simulink model "black_box_ex1_new"  (Simulink 7.3)
settings: Solver=VariableStepDiscrete  SolverMode=SingleTasking  StartTime=0.0  StopTime=500  RelTol=1e-3
undefined symbols (not defined in the file or in its folder): dfilt, xlipgetpartsetting
libraries: xbsIndex_r4 x12, xbsCopyrightNotice_r4 x1, dsparch4 x1, dspobslib x1, simulink x1
settings Model: Creator=alexc  LastModifiedBy=douangp
settings DataIOCC: SignalLoggingName=sigsOut
settings OptimizationCC: InitFltsAndDblsToZero=on
settings DebuggingCC: SaveWithParameterizedLinksMsg=none  SignalResolutionControl=TryResolveAllWithWarning  SolverPrmCheckMsg=none  MultiTaskDSMMsg=warning  MultiTaskCondExecSysMsg=none  StrictBusMsg=None
settings HardwareCC: TargetUnknown=on
settings RTWCC: IncludeERTFirstTime=on
settings GRTTargetCC: TargetFcnLib=ansi_tfl_tmw.mat

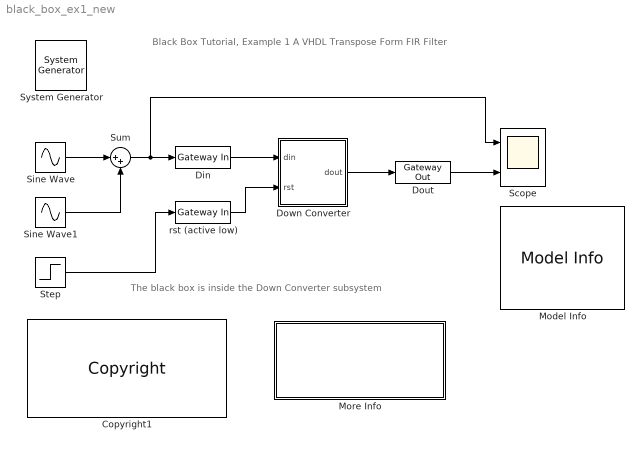
== system black_box_ex1_new ==
  note: Black Box Tutorial, Example 1
      | A VHDL Transpose Form FIR Filter
  note: The black box is inside the
      | Down Converter subsystem
  " System Generator" : xbsIndex_r4/ System Generator  Tag=genX  SystemSampleTime=-1  xilinxfamily=virtex6  part=xc6vlx240t  speed=-1  package=ff1156  synthesis_tool=XST  clock_wrapper=Clock Enables  directory=./netlist  testbench=off  simulink_period=1  sysclk_period=5  dcm_input_clock_period=100  incr_netlist=off  trim_vbits=Everywhere in SubSystem  dbl_ovrd=According to Block Masks  core_generation=According to Block Masks  run_coregen=off  deprecated_control=off  eval_field=0  block_type=sysgen
      settings: block_version=9.2.01
  Copyright1 : xbsCopyrightNotice_r4/Copyright  copyrighttext="Copyright (c) 2009  by  Xilinx, Inc. All rights reserved.<br><br>This file contains proprietary, confidential information of Xilinx, Inc., is distributed under licensefrom Xilinx, Inc., and may be used, copied and/or disclosed only pursuant to the terms of a valid licenseagreement with Xilinx, Inc. Xilinx hereby grants you a license to use this file solely for design,simulation, implementation and creation of design files limited to Xilinx devices or technologies. Use with non-Xilinx devices or technologies is expressly prohibited and immediately terminates your license unless covered by a separate agreement.<br><br>Xilinx is providing this design, code, or information \"as-is\" solely for use in developing programs and solutions for Xilinx devices, with no obligation on the part of Xilinx to provide support. By providingthis design, code, or information as one possible implementation of this feature, application or standard,Xilinx is making no representation that this implementation is free from any claims of infringement. Youare responsible for obtaining any rights you may require for your implementation. Xilinx expressly disclaimsany warranty whatsoever with respect to the adequacy of the implementation, including but not limited to anywarranties or representations that this implementation is free from claims of infringement, implied warrantiesof merchantability or fitness for a particular purpose.<br><br>Xilinx products are not intended for use in life support appliances, devices, or systems. Use in such applications is expressly prohibited.<br><br>Any modifications that are made to the Source Code are done at the user's sole risk and will be unsupported.<br><br>This copyright and support notice must be retained as part of this text at all times. (c) Copyright 1995-2009 Xilinx, Inc. All rights reserved."  block_type=copyright
      settings: block_version=10.1.00
      settings: infoedit=|
      | Copyright(C) 2008 by  Xilinx, Inc. All rights reserved.<br>
      | <br>
      | This file contains proprietary, confidential information of Xilinx, Inc., is distributed under license
      | from Xilinx, Inc., and may be used, copied and/or disclosed only pursuant to the terms of a valid license
      | agreement with Xilinx, Inc. Xilinx hereby grants you a license to use this file solely for design,
      | simulation, implementation and creation of design files limited to Xilinx devices or technologies. Use
      | with non-Xilinx devices or technologies is expressly prohibited and immediately terminates your license
      | unless covered by a separate agreement.<br>
      | <br>
      | Xilinx is providing this design, code, or information "as-is" solely for use in developing programs and
      | solutions for Xilinx devices, with no obligation on the part of Xilinx to provide support. By providing
      | this design, code, or information as one possible implementation of this feature, application or standard,
      | Xilinx is making no representation that this implementation is free from any claims of infringement. You
      | are responsible for obtaining any rights you may require for your implementation. Xilinx expressly disclaims
      | any warranty whatsoever with respect to the adequacy of the implementation, including but not limited to any
      | warranties or representations that this implementation is free from claims of infringement, implied warranties
      | of merchantability or fitness for a particular purpose.<br>
      | <br>
      | Xilinx products are not intended for use in life support appliances, devices, or systems. Use in such
      | applications is expressly prohibited.<br>
      | <br>
      | Any modifications that are made to the Source Code are done at the user's sole risk and will be unsupported.<br>
      | <br>
      | This copyright and support notice must be retained as part of this text at all times.
      | (c) Copyright 1995-2008 Xilinx, Inc. All rights reserved.
  Din : xbsIndex_r4/Gateway In  arith_type="Signed  (2's comp)"  n_bits=10  bin_pt=8  quantization="Round  (unbiased: +/- Inf)"  overflow=Saturate  period=1  dbl_ovrd=off  timing_constraint=None  locs_specified=off  LOCs={}  block_type=gatewayin
      settings: infoedit="Gateway in block.  Converts inputs of type Simulink integer, double and fixed point to  Xilinx fixed point type.<P><P>Hardware notes:  In hardware these blocks become top level input ports."  xl_area=[0, 0, 0, 0, 0, 0, 0]  block_version=VER_STRING_GOES_HERE
  Dout : xbsIndex_r4/Gateway Out  hdl_port=on  timing_constraint=None  locs_specified=off  LOCs={}  block_type=gatewayout
      settings: infoedit="Gateway out block.  Converts Xilinx fixed point inputs into ouputs of type Simulink integer, double, or fixed point.<P><P>Hardware notes:  In hardware these blocks become top level output ports or are discarded, depending on how they are configured."  xl_area=[0, 0, 0, 0, 0, 0, 0]  block_version=VER_STRING_GOES_HERE
  Down Converter : Subsystem
  Model Info : simulink/Model-Wide Utilities/Model Info  SystemSampleTime=-1  InitialBlockCM=None  BlockCM=None  Frame=on  DisplayStringWithTags=|  HorizontalTextAlignment=Left  LeftAlignmentValue=0.02  SourceBlockDiagram=black_box_ex1_new  TagMaxNumber=20
      | Model Info
      | Created by %<Created>
      | Modified by %<ModifiedBy>
      | Model version %<ModelVersion>
  More Info : Subsystem
      settings: OpenFcn=xlDoc('-book','sysgen', '-title', 'Black Box');
      mask Display: disp('Double click\n for System Generator\n documentation on\n related topics.')
  Scope : Scope  NumInputPorts=2
      settings: YMin=-2~-7000  YMax=2~7000
  Sine Wave : Sin  Amplitude=1  Bias=0  Frequency=2*pi*.31  Phase=0  Samples=10  SampleTime=1  Offset=0
  Sine Wave1 : Sin  Amplitude=1  Bias=0  Frequency=2*pi*.45  Phase=0  Samples=10  SampleTime=1  Offset=0
  Step : Step  SampleTime=1
  Sum : Sum  Inputs=|++  OutDataType=sfix(16)  OutScaling=2^0  SaturateOnIntegerOverflow=on
  rst (active low) : xbsIndex_r4/Gateway In  arith_type=Boolean  n_bits=10  bin_pt=8  quantization="Round  (unbiased: +/- Inf)"  overflow=Saturate  period=1  dbl_ovrd=off  timing_constraint=None  locs_specified=off  LOCs={}  block_type=gatewayin
      settings: infoedit="Gateway in block.  Converts inputs of type Simulink integer, double and fixed point to  Xilinx fixed point type.<P><P>Hardware notes:  In hardware these blocks become top level input ports."  xl_area=[0, 0, 0, 0, 0, 0, 0]  block_version=VER_STRING_GOES_HERE
  wires:
  Down Converter/1(dout) -> Dout/1
  Din/1 -> Down Converter/1(din)
  Dout/1 -> Scope/2
  Sine Wave/1 -> Sum/1
  Sine Wave1/1 -> Sum/2
  Sum/1 -> Din/1, Scope/1
  rst (active low)/1 -> Down Converter/2(rst)
  Step/1 -> rst (active low)/1

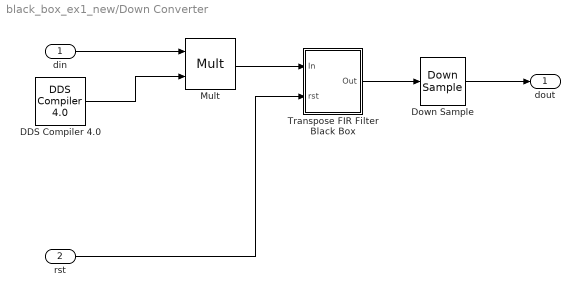
== system black_box_ex1_new/Down Converter ==
  din : Inport  OutDataType=sfix(16)  OutScaling=2^0
  rst : Inport  Port=2  OutDataType=sfix(16)  OutScaling=2^0
  "DDS Compiler 4.0 " : xbsIndex_r4/DDS Compiler 4.0   partspresent=Phase_Generator_and_SIN_COS_LUT  dds_clock_rate=100  channels=1  parameter_entry=System_Parameters  spurious_free_dynamic_range=50  frequency_resolution=0.4  noise_shaping=None  phase_width=28  output_width=6  output_selection=Sine  negative_sine=off  negative_cosine=off  amplitude_mode=Full_Range  memory_type=Auto  optimization_goal=Auto  dsp48_use=Minimal  latency_configuration=Auto  latency=2  has_phase_out=off  sclr_pin=off  clock_enable=off  rfd=off  rdy=off  channel_pin=off  explicit_period=on  period=1  phase_increment=Fixed  output_frequency1=30  output_frequency2=0  output_frequency3=0  output_frequency4=0  output_frequency5=0  output_frequency6=0  output_frequency7=0  output_frequency8=0  output_frequency9=0  output_frequency10=0  output_frequency11=0  output_frequency12=0  output_frequency13=0  output_frequency14=0  output_frequency15=0  output_frequency16=0  pinc1='0'  pinc2='0'  pinc3='0'  pinc4='0'  pinc5='0'  pinc6='0'  pinc7='0'  pinc8='0'  pinc9='0'  pinc10='0'  pinc11='0'  pinc12='0'  pinc13='0'  pinc14='0'  pinc15='0'  pinc16='0'  phase_offset=None  phase_offset_angles1=0  phase_offset_angles2=0  phase_offset_angles3=0  phase_offset_angles4=0  phase_offset_angles5=0  phase_offset_angles6=0  phase_offset_angles7=0  phase_offset_angles8=0  phase_offset_angles9=0  phase_offset_angles10=0  phase_offset_angles11=0  phase_offset_angles12=0  phase_offset_angles13=0  phase_offset_angles14=0  phase_offset_angles15=0  phase_offset_angles16=0  poff1='0'  poff2='0'  poff3='0'  poff4='0'  poff5='0'  poff6='0'  poff7='0'  poff8='0'  poff9='0'  poff10='0'  poff11='0'  poff12='0'  poff13='0'  poff14='0'  poff15='0'  poff16='0'  por_mode=false  gui_behaviour=Sysgen  ip_name=DDS Compiler  ip_version=4.0  dsptool_ready=true  wrapper_available=true  port_translation_map={ 'ce' => 'en', 'sclr' => 'rst' }  ipcore_xco_need_fpga_part=true  ipcore_fpga_part=xlipgetpartsetting(gcb, {'virtex4', 'xc4vsx35', '-10', 'ff668'})  ipcore_usecache=true  ipcore_useipmodelcache=true  ipcore_verbose=false  block_type=dds_compiler_v4_0
      settings: block_version=11.3
  Down Sample : xbsIndex_r4/Down Sample  sample_ratio=4  sample_phase="Last Value of Frame  (most efficient)"  en=off  latency=1  dbl_ovrd=off  block_type=dsamp
      settings: xl_area=[0, 0, 0, 0, 0, 0, 0]  block_version=VER_STRING_GOES_HERE
  Mult : xbsIndex_r4/Mult  precision=User Defined  arith_type="Signed  (2's comp)"  n_bits=12  bin_pt=9  quantization=Truncate  overflow=Wrap  en=off  latency=2  dbl_ovrd=off  use_behavioral_HDL=off  opt=Speed  use_embedded=on  optimum_pipeline=off  pipeline=on  use_rpm=off  placement_style=Rectangular shape  block_type=mult
      settings: infoedit=Multiplies two values.<P><P>Hardware notes: To use the internal pipeline stage of the dedicated multiplier you must select 'Pipeline to Greatest Extent Possible'.  xl_area=[0, 0, 0, 0, 0, 0, 0]  block_version=VER_STRING_GOES_HERE
  Transpose FIR Filter Black Box : Subsystem
  dout : Outport  OutDataType=sfix(16)  OutScaling=2^0
  wires:
  din/1 -> Mult/1
  Mult/1 -> Transpose FIR Filter Black Box/1(In)
  Transpose FIR Filter Black Box/1(Out) -> Down Sample/1
  "DDS Compiler 4.0 "/1 -> Mult/2
  Down Sample/1 -> dout/1
  rst/1 -> Transpose FIR Filter Black Box/2(rst)

== system black_box_ex1_new/More Info ==

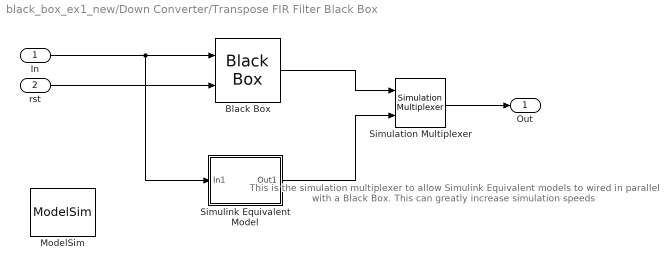
== system black_box_ex1_new/Down Converter/Transpose FIR Filter Black Box ==
  note: This is the simulation
      | multiplexer to allow
      | Simulink Equivalent
      | models to wired in parallel
      | with a Black Box. This
      | can greatly increase
      | simulation speeds
  In : Inport  OutDataType=sfix(16)  OutScaling=2^0
  rst : Inport  Port=2  OutDataType=sfix(16)  OutScaling=2^0
  Black Box : xbsIndex_r4/Black Box  init_code=transpose_fir_config  sim_method=ISE Simulator  engine_block=ModelSim  verbose=off  block_type=blackbox2
      settings: xl_area=[0, 0, 0, 0, 0, 0, 0]  block_version=VER_STRING_GOES_HERE
  ModelSim : xbsIndex_r4/ModelSim  dir=./modelsim  waveform=on  leave_open=on  skip_compile=off  use_unisim=off  custom_scripts=off  startup_timeout=40  block_type=hdlcosim
      settings: infoedit="Allows other blocks to schedule HDL co-simulation tasks.<P><P>Note that selecting the \"Skip Compilation\" when inappropriate can cause simulation errors and failures. Please refer to the block help for details."  block_version=VER_STRING_GOES_HERE
  Simulation Multiplexer : xbsIndex_r4/Simulation Multiplexer  sim_sel=2  hw_sel=1  block_type=simmux
      settings: infoedit="Distinguish input subsystems as \"simulation only\" and \"generation only\".  The input specified For Simulation will be used during Simulink simulation.  The input specified For Generation will be used during code generation.  This block will typically be used on the output of a HW Co-Simulation, Black Box, or ModelSim subsystem.<P><P>Hardware Notes: This block costs nothing."  block_version=VER_STRING_GOES_HERE
  Simulink Equivalent Model : Subsystem
  Out : Outport  OutDataType=sfix(16)  OutScaling=2^0
  wires:
  In/1 -> Simulink Equivalent Model/1(In1), Black Box/1
  Simulink Equivalent Model/1(Out1) -> Simulation Multiplexer/2
  Simulation Multiplexer/1 -> Out/1
  Black Box/1 -> Simulation Multiplexer/1
  rst/1 -> Black Box/2

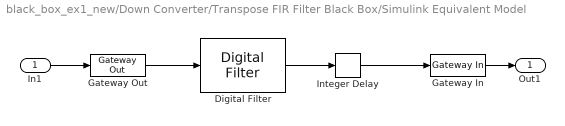
== system black_box_ex1_new/Down Converter/Transpose FIR Filter Black Box/Simulink Equivalent Model ==
  In1 : Inport  OutDataType=sfix(16)  OutScaling=2^0
  Digital Filter : dsparch4/Digital Filter  DialogController=dspdialog.DigitalFilter  DialogControllerArgs=DataTag1  TypePopup=FIR (all zeros)  IIRFiltStruct=Direct form II transposed  AllPoleFiltStruct=Direct form  FIRFiltStruct=Direct form  CoeffSource=Specify via dialog  NumCoeffs=[-38 -74 -109 -109 -37 140 435 827 1262 1663 1945 2047 1945 1663 1262 827 435 140 -37 -109 -109 -74 -38]  DenCoeffs=[1 0.1]  BiQuadCoeffs=[1 0.3 0.4 1 0.1 0.2]  LatticeCoeffs=[0.2 0.4]  denIgnore=on  FiltPerSampPopup=One filter per frame  IC=0  ICnum=0  ICden=0  roundingMode=Floor  overflowMode=off  ScaleValues=1  scaleValueFracLength=14  stageInFracLength=15  stageOutFracLength=15  FilterSource=Specify via dialog  dfiltObjectName=dfilt.dffir([1 2 1])
  Gateway In : xbsIndex_r4/Gateway In  arith_type="Signed  (2's comp)"  n_bits=26  bin_pt=12  quantization="Round  (unbiased: +/- Inf)"  overflow=Saturate  period=1  dbl_ovrd=off  timing_constraint=None  locs_specified=off  LOCs={}  block_type=gatewayin
      settings: infoedit="Gateway in block.  Converts inputs of type Simulink integer, double and fixed point to  Xilinx fixed point type.<P><P>Hardware notes:  In hardware these blocks become top level input ports."  xl_area=[0, 0, 0, 0, 0, 0, 0]  block_version=VER_STRING_GOES_HERE
  Gateway Out : xbsIndex_r4/Gateway Out  hdl_port=on  timing_constraint=None  locs_specified=off  LOCs={}  block_type=gatewayout
      settings: infoedit="Gateway out block.  Converts Xilinx fixed point inputs into ouputs of type Simulink integer, double, or fixed point.<P><P>Hardware notes:  In hardware these blocks become top level output ports or are discarded, depending on how they are configured."  xl_area=[0, 0, 0, 0, 0, 0, 0]  block_version=VER_STRING_GOES_HERE
  Integer Delay : dspobslib/Integer Delay  delay=1  ic=0  reset_popup=None
  Out1 : Outport  OutDataType=sfix(16)  OutScaling=2^0
  wires:
  Digital Filter/1 -> Integer Delay/1
  In1/1 -> Gateway Out/1
  Integer Delay/1 -> Gateway In/1
  Gateway Out/1 -> Digital Filter/1
  Gateway In/1 -> Out1/1
